simulink model "RoboBoat_SLAM_6_29"  (R2014a)
settings: Solver=FixedStepDiscrete  StartTime=0.0  StopTime=inf  FixedStep=.1  RelTol=1e-3
undefined symbols (not defined in the file): Com1, Com2, Com3, Com4, DiscIntNeverNeededParam, standard
libraries: xpcseriallib x29, visiontextngfix x25, simulink x21, slrtlib x7, speedgoatlib_IO102 x5, speedgoatlib x1
(part 4 of 6)

== system RoboBoat_SLAM_6_29/Main FSM/Obstacle Navigation1/GPS: Center/Approach ==
  Sensors : Inport
  RGB image : Inport  Port=2
  Enable : EnablePort
  Annotate Task : visiontextngfix/Insert Text  inputType=Obsolete  theText='GPS - Center: Approach - Distance: %f'  getTextLocFrom=Specify via dialog  textLoc=[10 70]  getTextColorFrom=Specify via dialog  textColor=[255 0 0]  getTextIntensityFrom=Specify via dialog  textIntensity=0  getTextOpacityFrom=Specify via dialog  textOpacity=1.0  dummyVar2=0  dummyVar3=0  dummyVar4=0  imagePorts=One multidimensional signal  isInputTransposed=off  fontFace=LucidaSansRegular  dummyVar1=0  blockFontSize=12  antiAliased=on
  Annotate Task2 : visiontextngfix/Insert Text  inputType=Obsolete  theText='Obst Nav Start'  getTextLocFrom=Specify via dialog  textLoc=[1 1]  getTextColorFrom=Specify via dialog  textColor=[0 0 0]  getTextIntensityFrom=Specify via dialog  textIntensity=0  getTextOpacityFrom=Specify via dialog  textOpacity=1.0  dummyVar2=0  dummyVar3=0  dummyVar4=0  imagePorts=One multidimensional signal  isInputTransposed=off  fontFace=LucidaSansRegular  dummyVar1=0  blockFontSize=12  antiAliased=on
  Bus Selector : BusSelector  OutputSignals=Serial In.GPS.latitude,Serial In.GPS.longitude
  Compare To Constant : simulink/Logic and Bit Operations/Compare To Constant  relop=<=  const=5  OutDataTypeStr=boolean
  Data Store Read : DataStoreRead  DataStoreName=obstNavStartGPS  SampleTime=0.1
  Data Type Conversion : DataTypeConversion  OutDataTypeStr=double
  Desired Heading and Distance : MATLAB Function  TreatAsAtomicUnit=on
  MATLAB Function : MATLAB Function  Commented=on  TreatAsAtomicUnit=on
  Output Heirarchy : Subsystem
  "Scope " : slrtlib/Displays and Logging/Scope   Commented=on  scopeno=1  scopetype=File  autostart=on  viewmode=Graphical redraw  formatstr='%15.6f'  grid=on  ylimits=[0,0]  nosamples=1200  noprepostsamples=0  interleave=1  triggermode=FreeRun  triggersignal=1  trigsignalfromport=off  triggerlevel=1  triggerslope=Either  triggerscope=1  triggersample=0  filename=ApprLog.dat  mode=Lazy  writesize=512  autorestart=off  dynamicfilemode=off  maxwritefilesize=512*1024^2
  Outputs : Outport
  wires:
  Sensors/1 -> Output Heirarchy/4(Sensors), Bus Selector/1  "Sensors"
  Data Store Read/1 -> Desired Heading and Distance/1(DesiredGPS)
  Bus Selector/1 -> Desired Heading and Distance/2(GPSLat)  "<latitude>"
  Bus Selector/2 -> Desired Heading and Distance/3(GPSLong)  "<longitude>"
  Desired Heading and Distance/2(DesiredHeading) -> Output Heirarchy/2(Desired Heading)
  Annotate Task/1 -> Output Heirarchy/3(Annotated Image)
  RGB image/1 -> Annotate Task2/1
  Output Heirarchy/1(Outputs) -> Outputs/1
  Annotate Task2/1 -> Annotate Task/1
  MATLAB Function/1(out) -> "Scope "/1
  Desired Heading and Distance/1(Distance) -> Compare To Constant/1, Annotate Task/2
  Data Type Conversion/1 -> Output Heirarchy/1(Finished)  "Task Finished"
  Compare To Constant/1 -> Data Type Conversion/1

== system RoboBoat_SLAM_6_29/Main FSM/Obstacle Navigation1/GPS: Center/Orient ==
  Sensors : Inport
  RGB image : Inport  Port=2
  Enable : EnablePort
  Annotate Task : visiontextngfix/Insert Text  inputType=Obsolete  theText='GPS - Center: Orient %f'  getTextLocFrom=Specify via dialog  textLoc=[10 70]  getTextColorFrom=Specify via dialog  textColor=[255 0 0]  getTextIntensityFrom=Specify via dialog  textIntensity=0  getTextOpacityFrom=Specify via dialog  textOpacity=1.0  dummyVar2=0  dummyVar3=0  dummyVar4=0  imagePorts=One multidimensional signal  isInputTransposed=off  fontFace=LucidaSansRegular  dummyVar1=0  blockFontSize=12  antiAliased=on
  Annotate Task1 : visiontextngfix/Insert Text  inputType=Obsolete  theText='Current Heading %f'  getTextLocFrom=Specify via dialog  textLoc=[10 40]  getTextColorFrom=Specify via dialog  textColor=[255 0 0]  getTextIntensityFrom=Specify via dialog  textIntensity=0  getTextOpacityFrom=Specify via dialog  textOpacity=1.0  dummyVar2=0  dummyVar3=0  dummyVar4=0  imagePorts=One multidimensional signal  isInputTransposed=off  fontFace=LucidaSansRegular  dummyVar1=0  blockFontSize=12  antiAliased=on
  Annotate Task2 : visiontextngfix/Insert Text  inputType=Obsolete  theText='Obst Nav Start'  getTextLocFrom=Specify via dialog  textLoc=[1 1]  getTextColorFrom=Specify via dialog  textColor=[0 0 0]  getTextIntensityFrom=Specify via dialog  textIntensity=0  getTextOpacityFrom=Specify via dialog  textOpacity=1.0  dummyVar2=0  dummyVar3=0  dummyVar4=0  imagePorts=One multidimensional signal  isInputTransposed=off  fontFace=LucidaSansRegular  dummyVar1=0  blockFontSize=12  antiAliased=on
  Bus Selector : BusSelector  OutputSignals=Serial In.GPS.latitude,Serial In.GPS.longitude,Serial In.Compass.Heading
  Data Store Read : DataStoreRead  DataStoreName=obstNavStartGPS  SampleTime=0.1
  Desired Heading : MATLAB Function  TreatAsAtomicUnit=on
  Output Heirarchy1 : Subsystem
  Within Range : MATLAB Function  TreatAsAtomicUnit=on
  Outputs : Outport
  Finished : Outport  Port=2
  wires:
  Sensors/1 -> Output Heirarchy1/3(Sensors), Bus Selector/1  "Sensors"
  Data Store Read/1 -> Desired Heading/1(DesiredGPS)
  Bus Selector/1 -> Desired Heading/2(GPSLat)  "<latitude>"
  Bus Selector/2 -> Desired Heading/3(GPSLong)  "<longitude>"
  Desired Heading/1(DesiredHeading) -> Output Heirarchy1/2(Desired Heading), Annotate Task/2, Within Range/1(DesiredHeading)
  Bus Selector/3 -> Annotate Task1/2, Within Range/2(Compass)  "<Heading>"
  Within Range/1(Finished) -> Finished/1
  RGB image/1 -> Annotate Task2/1
  Output Heirarchy1/1(Outputs) -> Outputs/1
  Annotate Task/1 -> Annotate Task1/1
  Annotate Task1/1 -> Output Heirarchy1/1(Annotated Image)
  Annotate Task2/1 -> Annotate Task/1

== system RoboBoat_SLAM_6_29/Main FSM/Obstacle Navigation1/GPS: Center/Output Reassign ==
  Outputs in : Inport
  Bus Assignment : BusAssignment  AssignedSignals=Task Finished
  Bus Selector : BusSelector  OutputSignals=Task Finished
  Constant : Constant  Value=0
  Outputs : Outport
  Finished : Outport  Port=2
  wires:
  Outputs in/1 -> Bus Assignment/1, Bus Selector/1
  Bus Selector/1 -> Finished/1  "<Task Finished>"
  Bus Assignment/1 -> Outputs/1
  Constant/1 -> Bus Assignment/2

== system RoboBoat_SLAM_6_29/Main FSM/Obstacle Navigation1/Obstacle Navigation/Dodge ==
  Sensors : Inport
  RGB image : Inport  Port=2
  Enable : EnablePort  ShowOutputPort=on
  Bus Selector1 : BusSelector  OutputSignals=Serial In.Compass.Heading,Serial In.Buoy Info.Distance,Serial In.Buoy Info.Angle
  Constant : Constant  Value=0
  Constant1 : Constant  Value=2
  Data Store Write : DataStoreWrite  DataStoreName=dodgeStart
  Discrete-Time Integrator : DiscreteIntegrator  SampleTime=0.1  ICPrevOutput=DiscIntNeverNeededParam  ICPrevScaledInput=DiscIntNeverNeededParam
  Insert Text : visiontextngfix/Insert Text  inputType=Obsolete  theText='Dodge'  getTextLocFrom=Specify via dialog  textLoc=[1 1]  getTextColorFrom=Specify via dialog  textColor=[0 0 0]  getTextIntensityFrom=Specify via dialog  textIntensity=0  getTextOpacityFrom=Specify via dialog  textOpacity=1.0  dummyVar2=0  dummyVar3=0  dummyVar4=0  imagePorts=One multidimensional signal  isInputTransposed=off  fontFace=LucidaSansRegular  dummyVar1=0  blockFontSize=12  antiAliased=on
  Insert Text1 : visiontextngfix/Insert Text  inputType=Obsolete  theText='Obstacle Distance: %f'  getTextLocFrom=Specify via dialog  textLoc=[10 70]  getTextColorFrom=Specify via dialog  textColor=[255 0 0]  getTextIntensityFrom=Specify via dialog  textIntensity=0  getTextOpacityFrom=Specify via dialog  textOpacity=1.0  dummyVar2=0  dummyVar3=0  dummyVar4=0  imagePorts=One multidimensional signal  isInputTransposed=off  fontFace=LucidaSansRegular  dummyVar1=0  blockFontSize=12  antiAliased=on
  Nav Logic : MATLAB Function  TreatAsAtomicUnit=on
  Output Heirarchy : Subsystem
  Unit Delay1 : UnitDelay  InitialCondition=1  SampleTime=-1
  Outputs : Outport
  Dodge Incomplete : Outport  Port=2
  wires:
  RGB image/1 -> Insert Text/1
  Sensors/1 -> Output Heirarchy/2(Sensors), Bus Selector1/1
  Bus Selector1/1 -> Nav Logic/1(CurrentHeading)  "<Heading>"
  Enable/1 -> Discrete-Time Integrator/1
  Discrete-Time Integrator/1 -> Nav Logic/4(Timer)
  Constant1/1 -> Nav Logic/5(Timeout)
  Nav Logic/4(DodgeIncomplete) -> Dodge Incomplete/1
  Insert Text/1 -> Insert Text1/1
  Nav Logic/1(ObstDist) -> Insert Text1/2
  Nav Logic/2(RPM) -> Output Heirarchy/3(RPM)
  Nav Logic/3(DesiredHeading) -> Output Heirarchy/4(Desired Heading)
  Output Heirarchy/1(Outputs) -> Outputs/1
  Constant/1 -> Unit Delay1/1
  Unit Delay1/1 -> Data Store Write/1
  Insert Text1/1 -> Output Heirarchy/1(Annotated Image)
  Bus Selector1/2 -> Nav Logic/2(Dist)  "<Distance>"
  Bus Selector1/3 -> Nav Logic/3(Ang)  "<Angle>"

== system RoboBoat_SLAM_6_29/Main FSM/Obstacle Navigation1/Obstacle Navigation/GPS: Bee Line ==
  Sensors : Inport
  RGB image : Inport  Port=2
  Enable : EnablePort
  Approach : Subsystem  TreatAsAtomicUnit=on
  Data Store Write : DataStoreWrite  DataStoreName=dodgeStart
  GPS Enabler : MATLAB Function  TreatAsAtomicUnit=on
  GPS Selector : MultiPortSwitch  Inputs=2
  Orient : Subsystem  TreatAsAtomicUnit=on
  Unit Delay : UnitDelay  SampleTime=-1
  Unit Delay1 : UnitDelay  SampleTime=-1
  Outputs : Outport
  wires:
  Sensors/1 -> Orient/1(Sensors), Approach/1(Sensors)
  GPS Enabler/2(OrientEnable) -> Orient/Enable
  GPS Enabler/3(ApproachEnable) -> Approach/Enable
  Orient/2(Finished) -> Unit Delay/1
  Orient/1(Outputs) -> GPS Selector/2
  Approach/1(Outputs) -> GPS Selector/3
  GPS Enabler/1(GPSMode) -> GPS Selector/1
  Unit Delay/1 -> GPS Enabler/1(Finished)
  RGB image/1 -> Orient/2(RGB image), Approach/2(RGB image)
  Approach/2(Dodge Start) -> Unit Delay1/1
  Unit Delay1/1 -> Data Store Write/1
  GPS Selector/1 -> Outputs/1

== system RoboBoat_SLAM_6_29/Main FSM/Obstacle Navigation1/Obstacle Navigation/Output Reassign ==
  Outputs in : Inport
  Bus Assignment : BusAssignment  AssignedSignals=Task Finished
  Bus Selector : BusSelector  OutputSignals=Task Finished
  Constant : Constant  Value=0
  Outputs : Outport
  Finished : Outport  Port=2
  wires:
  Outputs in/1 -> Bus Assignment/1, Bus Selector/1
  Bus Selector/1 -> Finished/1  "<Task Finished>"
  Bus Assignment/1 -> Outputs/1
  Constant/1 -> Bus Assignment/2

== system RoboBoat_SLAM_6_29/Main FSM/SLAM/Models for prediction/Model1 ==
  X : Inport
  Y : Inport  Port=2
  Psi : Inport  Port=3
  Nav Messages : Inport  Port=4
  Bus Creator : BusCreator  Inputs=3
  Bus Selector : BusSelector  OutputSignals=IMU.Velocity.u,IMU.Velocity.v,IMU.Rate of Turn.GyrZ,Thrust.PortPow,Thrust.StbdPow
  Model : ModelReference  ModelNameDialog=SeaCat_Dynamic_Model.slx  SimulationMode=Normal  ModelReferenceVersion=1.2137  CopyOfModelName=SeaCat_Dynamic_Model.slx  DefaultDataLogging=on
  No Azimuth : Constant  Value=0
  NEyaw : Outport
  wires:
  Nav Messages/1 -> Bus Selector/1
  X/1 -> Model/1
  Y/1 -> Model/2
  Psi/1 -> Model/3
  Bus Selector/1 -> Model/4  "<u>"
  Bus Selector/2 -> Model/5  "<v>"
  Bus Selector/3 -> Model/6  "<GyrZ>"
  Bus Selector/4 -> Model/7  "<PortPow>"
  Bus Selector/5 -> Model/9  "<StbdPow>"
  No Azimuth/1 -> Model/8, Model/10
  Model/1 -> Bus Creator/1  "N"
  Model/3 -> Bus Creator/3  "yaw"
  Model/2 -> Bus Creator/2  "E"
  Bus Creator/1 -> NEyaw/1

== system RoboBoat_SLAM_6_29/Main FSM/SLAM/Models for prediction/Model10 ==
  X : Inport
  Y : Inport  Port=2
  Psi : Inport  Port=3
  Nav Messages : Inport  Port=4
  Bus Creator : BusCreator  Inputs=3
  Bus Selector : BusSelector  OutputSignals=IMU.Velocity.u,IMU.Velocity.v,IMU.Rate of Turn.GyrZ,Thrust.PortPow,Thrust.StbdPow
  Model : ModelReference  ModelNameDialog=SeaCat_Dynamic_Model.slx  SimulationMode=Normal  ModelReferenceVersion=1.2137  CopyOfModelName=SeaCat_Dynamic_Model.slx  DefaultDataLogging=on
  No Azimuth : Constant  Value=0
  NEyaw : Outport
  wires:
  Nav Messages/1 -> Bus Selector/1
  X/1 -> Model/1
  Y/1 -> Model/2
  Psi/1 -> Model/3
  Bus Selector/1 -> Model/4  "<u>"
  Bus Selector/2 -> Model/5  "<v>"
  Bus Selector/3 -> Model/6  "<GyrZ>"
  Bus Selector/4 -> Model/7  "<PortPow>"
  Bus Selector/5 -> Model/9  "<StbdPow>"
  No Azimuth/1 -> Model/8, Model/10
  Model/1 -> Bus Creator/1  "N"
  Model/3 -> Bus Creator/3  "yaw"
  Model/2 -> Bus Creator/2  "E"
  Bus Creator/1 -> NEyaw/1

== system RoboBoat_SLAM_6_29/Main FSM/SLAM/Models for prediction/Model11 ==
  X : Inport
  Y : Inport  Port=2
  Psi : Inport  Port=3
  Nav Messages : Inport  Port=4
  Bus Creator : BusCreator  Inputs=3
  Bus Selector : BusSelector  OutputSignals=IMU.Velocity.u,IMU.Velocity.v,IMU.Rate of Turn.GyrZ,Thrust.PortPow,Thrust.StbdPow
  Model : ModelReference  ModelNameDialog=SeaCat_Dynamic_Model.slx  SimulationMode=Normal  ModelReferenceVersion=1.2137  CopyOfModelName=SeaCat_Dynamic_Model.slx  DefaultDataLogging=on
  No Azimuth : Constant  Value=0
  NEyaw : Outport
  wires:
  Nav Messages/1 -> Bus Selector/1
  X/1 -> Model/1
  Y/1 -> Model/2
  Psi/1 -> Model/3
  Bus Selector/1 -> Model/4  "<u>"
  Bus Selector/2 -> Model/5  "<v>"
  Bus Selector/3 -> Model/6  "<GyrZ>"
  Bus Selector/4 -> Model/7  "<PortPow>"
  Bus Selector/5 -> Model/9  "<StbdPow>"
  No Azimuth/1 -> Model/8, Model/10
  Model/1 -> Bus Creator/1  "N"
  Model/3 -> Bus Creator/3  "yaw"
  Model/2 -> Bus Creator/2  "E"
  Bus Creator/1 -> NEyaw/1

== system RoboBoat_SLAM_6_29/Main FSM/SLAM/Models for prediction/Model12 ==
  X : Inport
  Y : Inport  Port=2
  Psi : Inport  Port=3
  Nav Messages : Inport  Port=4
  Bus Creator : BusCreator  Inputs=3
  Bus Selector : BusSelector  OutputSignals=IMU.Velocity.u,IMU.Velocity.v,IMU.Rate of Turn.GyrZ,Thrust.PortPow,Thrust.StbdPow
  Model : ModelReference  ModelNameDialog=SeaCat_Dynamic_Model.slx  SimulationMode=Normal  ModelReferenceVersion=1.2137  CopyOfModelName=SeaCat_Dynamic_Model.slx  DefaultDataLogging=on
  No Azimuth : Constant  Value=0
  NEyaw : Outport
  wires:
  Nav Messages/1 -> Bus Selector/1
  X/1 -> Model/1
  Y/1 -> Model/2
  Psi/1 -> Model/3
  Bus Selector/1 -> Model/4  "<u>"
  Bus Selector/2 -> Model/5  "<v>"
  Bus Selector/3 -> Model/6  "<GyrZ>"
  Bus Selector/4 -> Model/7  "<PortPow>"
  Bus Selector/5 -> Model/9  "<StbdPow>"
  No Azimuth/1 -> Model/8, Model/10
  Model/1 -> Bus Creator/1  "N"
  Model/3 -> Bus Creator/3  "yaw"
  Model/2 -> Bus Creator/2  "E"
  Bus Creator/1 -> NEyaw/1

== system RoboBoat_SLAM_6_29/Main FSM/SLAM/Models for prediction/Model13 ==
  X : Inport
  Y : Inport  Port=2
  Psi : Inport  Port=3
  Nav Messages : Inport  Port=4
  Bus Creator : BusCreator  Inputs=3
  Bus Selector : BusSelector  OutputSignals=IMU.Velocity.u,IMU.Velocity.v,IMU.Rate of Turn.GyrZ,Thrust.PortPow,Thrust.StbdPow
  Model : ModelReference  ModelNameDialog=SeaCat_Dynamic_Model.slx  SimulationMode=Normal  ModelReferenceVersion=1.2137  CopyOfModelName=SeaCat_Dynamic_Model.slx  DefaultDataLogging=on
  No Azimuth : Constant  Value=0
  NEyaw : Outport
  wires:
  Nav Messages/1 -> Bus Selector/1
  X/1 -> Model/1
  Y/1 -> Model/2
  Psi/1 -> Model/3
  Bus Selector/1 -> Model/4  "<u>"
  Bus Selector/2 -> Model/5  "<v>"
  Bus Selector/3 -> Model/6  "<GyrZ>"
  Bus Selector/4 -> Model/7  "<PortPow>"
  Bus Selector/5 -> Model/9  "<StbdPow>"
  No Azimuth/1 -> Model/8, Model/10
  Model/1 -> Bus Creator/1  "N"
  Model/3 -> Bus Creator/3  "yaw"
  Model/2 -> Bus Creator/2  "E"
  Bus Creator/1 -> NEyaw/1

== system RoboBoat_SLAM_6_29/Main FSM/SLAM/Models for prediction/Model14 ==
  X : Inport
  Y : Inport  Port=2
  Psi : Inport  Port=3
  Nav Messages : Inport  Port=4
  Bus Creator : BusCreator  Inputs=3
  Bus Selector : BusSelector  OutputSignals=IMU.Velocity.u,IMU.Velocity.v,IMU.Rate of Turn.GyrZ,Thrust.PortPow,Thrust.StbdPow
  Model : ModelReference  ModelNameDialog=SeaCat_Dynamic_Model.slx  SimulationMode=Normal  ModelReferenceVersion=1.2137  CopyOfModelName=SeaCat_Dynamic_Model.slx  DefaultDataLogging=on
  No Azimuth : Constant  Value=0
  NEyaw : Outport
  wires:
  Nav Messages/1 -> Bus Selector/1
  X/1 -> Model/1
  Y/1 -> Model/2
  Psi/1 -> Model/3
  Bus Selector/1 -> Model/4  "<u>"
  Bus Selector/2 -> Model/5  "<v>"
  Bus Selector/3 -> Model/6  "<GyrZ>"
  Bus Selector/4 -> Model/7  "<PortPow>"
  Bus Selector/5 -> Model/9  "<StbdPow>"
  No Azimuth/1 -> Model/8, Model/10
  Model/1 -> Bus Creator/1  "N"
  Model/3 -> Bus Creator/3  "yaw"
  Model/2 -> Bus Creator/2  "E"
  Bus Creator/1 -> NEyaw/1

== system RoboBoat_SLAM_6_29/Main FSM/SLAM/Models for prediction/Model15 ==
  X : Inport
  Y : Inport  Port=2
  Psi : Inport  Port=3
  Nav Messages : Inport  Port=4
  Bus Creator : BusCreator  Inputs=3
  Bus Selector : BusSelector  OutputSignals=IMU.Velocity.u,IMU.Velocity.v,IMU.Rate of Turn.GyrZ,Thrust.PortPow,Thrust.StbdPow
  Model : ModelReference  ModelNameDialog=SeaCat_Dynamic_Model.slx  SimulationMode=Normal  ModelReferenceVersion=1.2137  CopyOfModelName=SeaCat_Dynamic_Model.slx  DefaultDataLogging=on
  No Azimuth : Constant  Value=0
  NEyaw : Outport
  wires:
  Nav Messages/1 -> Bus Selector/1
  X/1 -> Model/1
  Y/1 -> Model/2
  Psi/1 -> Model/3
  Bus Selector/1 -> Model/4  "<u>"
  Bus Selector/2 -> Model/5  "<v>"
  Bus Selector/3 -> Model/6  "<GyrZ>"
  Bus Selector/4 -> Model/7  "<PortPow>"
  Bus Selector/5 -> Model/9  "<StbdPow>"
  No Azimuth/1 -> Model/8, Model/10
  Model/1 -> Bus Creator/1  "N"
  Model/3 -> Bus Creator/3  "yaw"
  Model/2 -> Bus Creator/2  "E"
  Bus Creator/1 -> NEyaw/1

== system RoboBoat_SLAM_6_29/Main FSM/SLAM/Models for prediction/Model16 ==
  X : Inport
  Y : Inport  Port=2
  Psi : Inport  Port=3
  Nav Messages : Inport  Port=4
  Bus Creator : BusCreator  Inputs=3
  Bus Selector : BusSelector  OutputSignals=IMU.Velocity.u,IMU.Velocity.v,IMU.Rate of Turn.GyrZ,Thrust.PortPow,Thrust.StbdPow
  Model : ModelReference  ModelNameDialog=SeaCat_Dynamic_Model.slx  SimulationMode=Normal  ModelReferenceVersion=1.2137  CopyOfModelName=SeaCat_Dynamic_Model.slx  DefaultDataLogging=on
  No Azimuth : Constant  Value=0
  NEyaw : Outport
  wires:
  Nav Messages/1 -> Bus Selector/1
  X/1 -> Model/1
  Y/1 -> Model/2
  Psi/1 -> Model/3
  Bus Selector/1 -> Model/4  "<u>"
  Bus Selector/2 -> Model/5  "<v>"
  Bus Selector/3 -> Model/6  "<GyrZ>"
  Bus Selector/4 -> Model/7  "<PortPow>"
  Bus Selector/5 -> Model/9  "<StbdPow>"
  No Azimuth/1 -> Model/8, Model/10
  Model/1 -> Bus Creator/1  "N"
  Model/3 -> Bus Creator/3  "yaw"
  Model/2 -> Bus Creator/2  "E"
  Bus Creator/1 -> NEyaw/1

== system RoboBoat_SLAM_6_29/Main FSM/SLAM/Models for prediction/Model17 ==
  X : Inport
  Y : Inport  Port=2
  Psi : Inport  Port=3
  Nav Messages : Inport  Port=4
  Bus Creator : BusCreator  Inputs=3
  Bus Selector : BusSelector  OutputSignals=IMU.Velocity.u,IMU.Velocity.v,IMU.Rate of Turn.GyrZ,Thrust.PortPow,Thrust.StbdPow
  Model : ModelReference  ModelNameDialog=SeaCat_Dynamic_Model.slx  SimulationMode=Normal  ModelReferenceVersion=1.2137  CopyOfModelName=SeaCat_Dynamic_Model.slx  DefaultDataLogging=on
  No Azimuth : Constant  Value=0
  NEyaw : Outport
  wires:
  Nav Messages/1 -> Bus Selector/1
  X/1 -> Model/1
  Y/1 -> Model/2
  Psi/1 -> Model/3
  Bus Selector/1 -> Model/4  "<u>"
  Bus Selector/2 -> Model/5  "<v>"
  Bus Selector/3 -> Model/6  "<GyrZ>"
  Bus Selector/4 -> Model/7  "<PortPow>"
  Bus Selector/5 -> Model/9  "<StbdPow>"
  No Azimuth/1 -> Model/8, Model/10
  Model/1 -> Bus Creator/1  "N"
  Model/3 -> Bus Creator/3  "yaw"
  Model/2 -> Bus Creator/2  "E"
  Bus Creator/1 -> NEyaw/1

== system RoboBoat_SLAM_6_29/Main FSM/SLAM/Models for prediction/Model18 ==
  X : Inport
  Y : Inport  Port=2
  Psi : Inport  Port=3
  Nav Messages : Inport  Port=4
  Bus Creator : BusCreator  Inputs=3
  Bus Selector : BusSelector  OutputSignals=IMU.Velocity.u,IMU.Velocity.v,IMU.Rate of Turn.GyrZ,Thrust.PortPow,Thrust.StbdPow
  Model : ModelReference  ModelNameDialog=SeaCat_Dynamic_Model.slx  SimulationMode=Normal  ModelReferenceVersion=1.2137  CopyOfModelName=SeaCat_Dynamic_Model.slx  DefaultDataLogging=on
  No Azimuth : Constant  Value=0
  NEyaw : Outport
  wires:
  Nav Messages/1 -> Bus Selector/1
  X/1 -> Model/1
  Y/1 -> Model/2
  Psi/1 -> Model/3
  Bus Selector/1 -> Model/4  "<u>"
  Bus Selector/2 -> Model/5  "<v>"
  Bus Selector/3 -> Model/6  "<GyrZ>"
  Bus Selector/4 -> Model/7  "<PortPow>"
  Bus Selector/5 -> Model/9  "<StbdPow>"
  No Azimuth/1 -> Model/8, Model/10
  Model/1 -> Bus Creator/1  "N"
  Model/3 -> Bus Creator/3  "yaw"
  Model/2 -> Bus Creator/2  "E"
  Bus Creator/1 -> NEyaw/1

== system RoboBoat_SLAM_6_29/Main FSM/SLAM/Models for prediction/Model19 ==
  X : Inport
  Y : Inport  Port=2
  Psi : Inport  Port=3
  Nav Messages : Inport  Port=4
  Bus Creator : BusCreator  Inputs=3
  Bus Selector : BusSelector  OutputSignals=IMU.Velocity.u,IMU.Velocity.v,IMU.Rate of Turn.GyrZ,Thrust.PortPow,Thrust.StbdPow
  Model : ModelReference  ModelNameDialog=SeaCat_Dynamic_Model.slx  SimulationMode=Normal  ModelReferenceVersion=1.2137  CopyOfModelName=SeaCat_Dynamic_Model.slx  DefaultDataLogging=on
  No Azimuth : Constant  Value=0
  NEyaw : Outport
  wires:
  Nav Messages/1 -> Bus Selector/1
  X/1 -> Model/1
  Y/1 -> Model/2
  Psi/1 -> Model/3
  Bus Selector/1 -> Model/4  "<u>"
  Bus Selector/2 -> Model/5  "<v>"
  Bus Selector/3 -> Model/6  "<GyrZ>"
  Bus Selector/4 -> Model/7  "<PortPow>"
  Bus Selector/5 -> Model/9  "<StbdPow>"
  No Azimuth/1 -> Model/8, Model/10
  Model/1 -> Bus Creator/1  "N"
  Model/3 -> Bus Creator/3  "yaw"
  Model/2 -> Bus Creator/2  "E"
  Bus Creator/1 -> NEyaw/1

== system RoboBoat_SLAM_6_29/Main FSM/SLAM/Models for prediction/Model2 ==
  X : Inport
  Y : Inport  Port=2
  Psi : Inport  Port=3
  Nav Messages : Inport  Port=4
  Bus Creator : BusCreator  Inputs=3
  Bus Selector : BusSelector  OutputSignals=IMU.Velocity.u,IMU.Velocity.v,IMU.Rate of Turn.GyrZ,Thrust.PortPow,Thrust.StbdPow
  Model : ModelReference  ModelNameDialog=SeaCat_Dynamic_Model.slx  SimulationMode=Normal  ModelReferenceVersion=1.2137  CopyOfModelName=SeaCat_Dynamic_Model.slx  DefaultDataLogging=on
  No Azimuth : Constant  Value=0
  NEyaw : Outport
  wires:
  Nav Messages/1 -> Bus Selector/1
  X/1 -> Model/1
  Y/1 -> Model/2
  Psi/1 -> Model/3
  Bus Selector/1 -> Model/4  "<u>"
  Bus Selector/2 -> Model/5  "<v>"
  Bus Selector/3 -> Model/6  "<GyrZ>"
  Bus Selector/4 -> Model/7  "<PortPow>"
  Bus Selector/5 -> Model/9  "<StbdPow>"
  No Azimuth/1 -> Model/8, Model/10
  Model/1 -> Bus Creator/1  "N"
  Model/3 -> Bus Creator/3  "yaw"
  Model/2 -> Bus Creator/2  "E"
  Bus Creator/1 -> NEyaw/1

== system RoboBoat_SLAM_6_29/Main FSM/SLAM/Models for prediction/Model20 ==
  X : Inport
  Y : Inport  Port=2
  Psi : Inport  Port=3
  Nav Messages : Inport  Port=4
  Bus Creator : BusCreator  Inputs=3
  Bus Selector : BusSelector  OutputSignals=IMU.Velocity.u,IMU.Velocity.v,IMU.Rate of Turn.GyrZ,Thrust.PortPow,Thrust.StbdPow
  Model : ModelReference  ModelNameDialog=SeaCat_Dynamic_Model.slx  SimulationMode=Normal  ModelReferenceVersion=1.2137  CopyOfModelName=SeaCat_Dynamic_Model.slx  DefaultDataLogging=on
  No Azimuth : Constant  Value=0
  NEyaw : Outport
  wires:
  Nav Messages/1 -> Bus Selector/1
  X/1 -> Model/1
  Y/1 -> Model/2
  Psi/1 -> Model/3
  Bus Selector/1 -> Model/4  "<u>"
  Bus Selector/2 -> Model/5  "<v>"
  Bus Selector/3 -> Model/6  "<GyrZ>"
  Bus Selector/4 -> Model/7  "<PortPow>"
  Bus Selector/5 -> Model/9  "<StbdPow>"
  No Azimuth/1 -> Model/8, Model/10
  Model/1 -> Bus Creator/1  "N"
  Model/3 -> Bus Creator/3  "yaw"
  Model/2 -> Bus Creator/2  "E"
  Bus Creator/1 -> NEyaw/1

== system RoboBoat_SLAM_6_29/Main FSM/SLAM/Models for prediction/Model21 ==
  X : Inport
  Y : Inport  Port=2
  Psi : Inport  Port=3
  Nav Messages : Inport  Port=4
  Bus Creator : BusCreator  Inputs=3
  Bus Selector : BusSelector  OutputSignals=IMU.Velocity.u,IMU.Velocity.v,IMU.Rate of Turn.GyrZ,Thrust.PortPow,Thrust.StbdPow
  Model : ModelReference  ModelNameDialog=SeaCat_Dynamic_Model.slx  SimulationMode=Normal  ModelReferenceVersion=1.2137  CopyOfModelName=SeaCat_Dynamic_Model.slx  DefaultDataLogging=on
  No Azimuth : Constant  Value=0
  NEyaw : Outport
  wires:
  Nav Messages/1 -> Bus Selector/1
  X/1 -> Model/1
  Y/1 -> Model/2
  Psi/1 -> Model/3
  Bus Selector/1 -> Model/4  "<u>"
  Bus Selector/2 -> Model/5  "<v>"
  Bus Selector/3 -> Model/6  "<GyrZ>"
  Bus Selector/4 -> Model/7  "<PortPow>"
  Bus Selector/5 -> Model/9  "<StbdPow>"
  No Azimuth/1 -> Model/8, Model/10
  Model/1 -> Bus Creator/1  "N"
  Model/3 -> Bus Creator/3  "yaw"
  Model/2 -> Bus Creator/2  "E"
  Bus Creator/1 -> NEyaw/1

== system RoboBoat_SLAM_6_29/Main FSM/SLAM/Models for prediction/Model22 ==
  X : Inport
  Y : Inport  Port=2
  Psi : Inport  Port=3
  Nav Messages : Inport  Port=4
  Bus Creator : BusCreator  Inputs=3
  Bus Selector : BusSelector  OutputSignals=IMU.Velocity.u,IMU.Velocity.v,IMU.Rate of Turn.GyrZ,Thrust.PortPow,Thrust.StbdPow
  Model : ModelReference  ModelNameDialog=SeaCat_Dynamic_Model.slx  SimulationMode=Normal  ModelReferenceVersion=1.2137  CopyOfModelName=SeaCat_Dynamic_Model.slx  DefaultDataLogging=on
  No Azimuth : Constant  Value=0
  NEyaw : Outport
  wires:
  Nav Messages/1 -> Bus Selector/1
  X/1 -> Model/1
  Y/1 -> Model/2
  Psi/1 -> Model/3
  Bus Selector/1 -> Model/4  "<u>"
  Bus Selector/2 -> Model/5  "<v>"
  Bus Selector/3 -> Model/6  "<GyrZ>"
  Bus Selector/4 -> Model/7  "<PortPow>"
  Bus Selector/5 -> Model/9  "<StbdPow>"
  No Azimuth/1 -> Model/8, Model/10
  Model/1 -> Bus Creator/1  "N"
  Model/3 -> Bus Creator/3  "yaw"
  Model/2 -> Bus Creator/2  "E"
  Bus Creator/1 -> NEyaw/1

== system RoboBoat_SLAM_6_29/Main FSM/SLAM/Models for prediction/Model23 ==
  X : Inport
  Y : Inport  Port=2
  Psi : Inport  Port=3
  Nav Messages : Inport  Port=4
  Bus Creator : BusCreator  Inputs=3
  Bus Selector : BusSelector  OutputSignals=IMU.Velocity.u,IMU.Velocity.v,IMU.Rate of Turn.GyrZ,Thrust.PortPow,Thrust.StbdPow
  Model : ModelReference  ModelNameDialog=SeaCat_Dynamic_Model.slx  SimulationMode=Normal  ModelReferenceVersion=1.2137  CopyOfModelName=SeaCat_Dynamic_Model.slx  DefaultDataLogging=on
  No Azimuth : Constant  Value=0
  NEyaw : Outport
  wires:
  Nav Messages/1 -> Bus Selector/1
  X/1 -> Model/1
  Y/1 -> Model/2
  Psi/1 -> Model/3
  Bus Selector/1 -> Model/4  "<u>"
  Bus Selector/2 -> Model/5  "<v>"
  Bus Selector/3 -> Model/6  "<GyrZ>"
  Bus Selector/4 -> Model/7  "<PortPow>"
  Bus Selector/5 -> Model/9  "<StbdPow>"
  No Azimuth/1 -> Model/8, Model/10
  Model/1 -> Bus Creator/1  "N"
  Model/3 -> Bus Creator/3  "yaw"
  Model/2 -> Bus Creator/2  "E"
  Bus Creator/1 -> NEyaw/1

== system RoboBoat_SLAM_6_29/Main FSM/SLAM/Models for prediction/Model24 ==
  X : Inport
  Y : Inport  Port=2
  Psi : Inport  Port=3
  Nav Messages : Inport  Port=4
  Bus Creator : BusCreator  Inputs=3
  Bus Selector : BusSelector  OutputSignals=IMU.Velocity.u,IMU.Velocity.v,IMU.Rate of Turn.GyrZ,Thrust.PortPow,Thrust.StbdPow
  Model : ModelReference  ModelNameDialog=SeaCat_Dynamic_Model.slx  SimulationMode=Normal  ModelReferenceVersion=1.2137  CopyOfModelName=SeaCat_Dynamic_Model.slx  DefaultDataLogging=on
  No Azimuth : Constant  Value=0
  NEyaw : Outport
  wires:
  Nav Messages/1 -> Bus Selector/1
  X/1 -> Model/1
  Y/1 -> Model/2
  Psi/1 -> Model/3
  Bus Selector/1 -> Model/4  "<u>"
  Bus Selector/2 -> Model/5  "<v>"
  Bus Selector/3 -> Model/6  "<GyrZ>"
  Bus Selector/4 -> Model/7  "<PortPow>"
  Bus Selector/5 -> Model/9  "<StbdPow>"
  No Azimuth/1 -> Model/8, Model/10
  Model/1 -> Bus Creator/1  "N"
  Model/3 -> Bus Creator/3  "yaw"
  Model/2 -> Bus Creator/2  "E"
  Bus Creator/1 -> NEyaw/1

== system RoboBoat_SLAM_6_29/Main FSM/SLAM/Models for prediction/Model25 ==
  X : Inport
  Y : Inport  Port=2
  Psi : Inport  Port=3
  Nav Messages : Inport  Port=4
  Bus Creator : BusCreator  Inputs=3
  Bus Selector : BusSelector  OutputSignals=IMU.Velocity.u,IMU.Velocity.v,IMU.Rate of Turn.GyrZ,Thrust.PortPow,Thrust.StbdPow
  Model : ModelReference  ModelNameDialog=SeaCat_Dynamic_Model.slx  SimulationMode=Normal  ModelReferenceVersion=1.2137  CopyOfModelName=SeaCat_Dynamic_Model.slx  DefaultDataLogging=on
  No Azimuth : Constant  Value=0
  NEyaw : Outport
  wires:
  Nav Messages/1 -> Bus Selector/1
  X/1 -> Model/1
  Y/1 -> Model/2
  Psi/1 -> Model/3
  Bus Selector/1 -> Model/4  "<u>"
  Bus Selector/2 -> Model/5  "<v>"
  Bus Selector/3 -> Model/6  "<GyrZ>"
  Bus Selector/4 -> Model/7  "<PortPow>"
  Bus Selector/5 -> Model/9  "<StbdPow>"
  No Azimuth/1 -> Model/8, Model/10
  Model/1 -> Bus Creator/1  "N"
  Model/3 -> Bus Creator/3  "yaw"
  Model/2 -> Bus Creator/2  "E"
  Bus Creator/1 -> NEyaw/1

== system RoboBoat_SLAM_6_29/Main FSM/SLAM/Models for prediction/Model26 ==
  X : Inport
  Y : Inport  Port=2
  Psi : Inport  Port=3
  Nav Messages : Inport  Port=4
  Bus Creator : BusCreator  Inputs=3
  Bus Selector : BusSelector  OutputSignals=IMU.Velocity.u,IMU.Velocity.v,IMU.Rate of Turn.GyrZ,Thrust.PortPow,Thrust.StbdPow
  Model : ModelReference  ModelNameDialog=SeaCat_Dynamic_Model.slx  SimulationMode=Normal  ModelReferenceVersion=1.2137  CopyOfModelName=SeaCat_Dynamic_Model.slx  DefaultDataLogging=on
  No Azimuth : Constant  Value=0
  NEyaw : Outport
  wires:
  Nav Messages/1 -> Bus Selector/1
  X/1 -> Model/1
  Y/1 -> Model/2
  Psi/1 -> Model/3
  Bus Selector/1 -> Model/4  "<u>"
  Bus Selector/2 -> Model/5  "<v>"
  Bus Selector/3 -> Model/6  "<GyrZ>"
  Bus Selector/4 -> Model/7  "<PortPow>"
  Bus Selector/5 -> Model/9  "<StbdPow>"
  No Azimuth/1 -> Model/8, Model/10
  Model/1 -> Bus Creator/1  "N"
  Model/3 -> Bus Creator/3  "yaw"
  Model/2 -> Bus Creator/2  "E"
  Bus Creator/1 -> NEyaw/1

== system RoboBoat_SLAM_6_29/Main FSM/SLAM/Models for prediction/Model27 ==
  X : Inport
  Y : Inport  Port=2
  Psi : Inport  Port=3
  Nav Messages : Inport  Port=4
  Bus Creator : BusCreator  Inputs=3
  Bus Selector : BusSelector  OutputSignals=IMU.Velocity.u,IMU.Velocity.v,IMU.Rate of Turn.GyrZ,Thrust.PortPow,Thrust.StbdPow
  Model : ModelReference  ModelNameDialog=SeaCat_Dynamic_Model.slx  SimulationMode=Normal  ModelReferenceVersion=1.2137  CopyOfModelName=SeaCat_Dynamic_Model.slx  DefaultDataLogging=on
  No Azimuth : Constant  Value=0
  NEyaw : Outport
  wires:
  Nav Messages/1 -> Bus Selector/1
  X/1 -> Model/1
  Y/1 -> Model/2
  Psi/1 -> Model/3
  Bus Selector/1 -> Model/4  "<u>"
  Bus Selector/2 -> Model/5  "<v>"
  Bus Selector/3 -> Model/6  "<GyrZ>"
  Bus Selector/4 -> Model/7  "<PortPow>"
  Bus Selector/5 -> Model/9  "<StbdPow>"
  No Azimuth/1 -> Model/8, Model/10
  Model/1 -> Bus Creator/1  "N"
  Model/3 -> Bus Creator/3  "yaw"
  Model/2 -> Bus Creator/2  "E"
  Bus Creator/1 -> NEyaw/1

== system RoboBoat_SLAM_6_29/Main FSM/SLAM/Models for prediction/Model28 ==
  X : Inport
  Y : Inport  Port=2
  Psi : Inport  Port=3
  Nav Messages : Inport  Port=4
  Bus Creator : BusCreator  Inputs=3
  Bus Selector : BusSelector  OutputSignals=IMU.Velocity.u,IMU.Velocity.v,IMU.Rate of Turn.GyrZ,Thrust.PortPow,Thrust.StbdPow
  Model : ModelReference  ModelNameDialog=SeaCat_Dynamic_Model.slx  SimulationMode=Normal  ModelReferenceVersion=1.2137  CopyOfModelName=SeaCat_Dynamic_Model.slx  DefaultDataLogging=on
  No Azimuth : Constant  Value=0
  NEyaw : Outport
  wires:
  Nav Messages/1 -> Bus Selector/1
  X/1 -> Model/1
  Y/1 -> Model/2
  Psi/1 -> Model/3
  Bus Selector/1 -> Model/4  "<u>"
  Bus Selector/2 -> Model/5  "<v>"
  Bus Selector/3 -> Model/6  "<GyrZ>"
  Bus Selector/4 -> Model/7  "<PortPow>"
  Bus Selector/5 -> Model/9  "<StbdPow>"
  No Azimuth/1 -> Model/8, Model/10
  Model/1 -> Bus Creator/1  "N"
  Model/3 -> Bus Creator/3  "yaw"
  Model/2 -> Bus Creator/2  "E"
  Bus Creator/1 -> NEyaw/1

== system RoboBoat_SLAM_6_29/Main FSM/SLAM/Models for prediction/Model29 ==
  X : Inport
  Y : Inport  Port=2
  Psi : Inport  Port=3
  Nav Messages : Inport  Port=4
  Bus Creator : BusCreator  Inputs=3
  Bus Selector : BusSelector  OutputSignals=IMU.Velocity.u,IMU.Velocity.v,IMU.Rate of Turn.GyrZ,Thrust.PortPow,Thrust.StbdPow
  Model : ModelReference  ModelNameDialog=SeaCat_Dynamic_Model.slx  SimulationMode=Normal  ModelReferenceVersion=1.2137  CopyOfModelName=SeaCat_Dynamic_Model.slx  DefaultDataLogging=on
  No Azimuth : Constant  Value=0
  NEyaw : Outport
  wires:
  Nav Messages/1 -> Bus Selector/1
  X/1 -> Model/1
  Y/1 -> Model/2
  Psi/1 -> Model/3
  Bus Selector/1 -> Model/4  "<u>"
  Bus Selector/2 -> Model/5  "<v>"
  Bus Selector/3 -> Model/6  "<GyrZ>"
  Bus Selector/4 -> Model/7  "<PortPow>"
  Bus Selector/5 -> Model/9  "<StbdPow>"
  No Azimuth/1 -> Model/8, Model/10
  Model/1 -> Bus Creator/1  "N"
  Model/3 -> Bus Creator/3  "yaw"
  Model/2 -> Bus Creator/2  "E"
  Bus Creator/1 -> NEyaw/1

== system RoboBoat_SLAM_6_29/Main FSM/SLAM/Models for prediction/Model3 ==
  X : Inport
  Y : Inport  Port=2
  Psi : Inport  Port=3
  Nav Messages : Inport  Port=4
  Bus Creator : BusCreator  Inputs=3
  Bus Selector : BusSelector  OutputSignals=IMU.Velocity.u,IMU.Velocity.v,IMU.Rate of Turn.GyrZ,Thrust.PortPow,Thrust.StbdPow
  Model : ModelReference  ModelNameDialog=SeaCat_Dynamic_Model.slx  SimulationMode=Normal  ModelReferenceVersion=1.2137  CopyOfModelName=SeaCat_Dynamic_Model.slx  DefaultDataLogging=on
  No Azimuth : Constant  Value=0
  NEyaw : Outport
  wires:
  Nav Messages/1 -> Bus Selector/1
  X/1 -> Model/1
  Y/1 -> Model/2
  Psi/1 -> Model/3
  Bus Selector/1 -> Model/4  "<u>"
  Bus Selector/2 -> Model/5  "<v>"
  Bus Selector/3 -> Model/6  "<GyrZ>"
  Bus Selector/4 -> Model/7  "<PortPow>"
  Bus Selector/5 -> Model/9  "<StbdPow>"
  No Azimuth/1 -> Model/8, Model/10
  Model/1 -> Bus Creator/1  "N"
  Model/3 -> Bus Creator/3  "yaw"
  Model/2 -> Bus Creator/2  "E"
  Bus Creator/1 -> NEyaw/1

== system RoboBoat_SLAM_6_29/Main FSM/SLAM/Models for prediction/Model30 ==
  X : Inport
  Y : Inport  Port=2
  Psi : Inport  Port=3
  Nav Messages : Inport  Port=4
  Bus Creator : BusCreator  Inputs=3
  Bus Selector : BusSelector  OutputSignals=IMU.Velocity.u,IMU.Velocity.v,IMU.Rate of Turn.GyrZ,Thrust.PortPow,Thrust.StbdPow
  Model : ModelReference  ModelNameDialog=SeaCat_Dynamic_Model.slx  SimulationMode=Normal  ModelReferenceVersion=1.2137  CopyOfModelName=SeaCat_Dynamic_Model.slx  DefaultDataLogging=on
  No Azimuth : Constant  Value=0
  NEyaw : Outport
  wires:
  Nav Messages/1 -> Bus Selector/1
  X/1 -> Model/1
  Y/1 -> Model/2
  Psi/1 -> Model/3
  Bus Selector/1 -> Model/4  "<u>"
  Bus Selector/2 -> Model/5  "<v>"
  Bus Selector/3 -> Model/6  "<GyrZ>"
  Bus Selector/4 -> Model/7  "<PortPow>"
  Bus Selector/5 -> Model/9  "<StbdPow>"
  No Azimuth/1 -> Model/8, Model/10
  Model/1 -> Bus Creator/1  "N"
  Model/3 -> Bus Creator/3  "yaw"
  Model/2 -> Bus Creator/2  "E"
  Bus Creator/1 -> NEyaw/1

== system RoboBoat_SLAM_6_29/Main FSM/SLAM/Models for prediction/Model31 ==
  X : Inport
  Y : Inport  Port=2
  Psi : Inport  Port=3
  Nav Messages : Inport  Port=4
  Bus Creator : BusCreator  Inputs=3
  Bus Selector : BusSelector  OutputSignals=IMU.Velocity.u,IMU.Velocity.v,IMU.Rate of Turn.GyrZ,Thrust.PortPow,Thrust.StbdPow
  Model : ModelReference  ModelNameDialog=SeaCat_Dynamic_Model.slx  SimulationMode=Normal  ModelReferenceVersion=1.2137  CopyOfModelName=SeaCat_Dynamic_Model.slx  DefaultDataLogging=on
  No Azimuth : Constant  Value=0
  NEyaw : Outport
  wires:
  Nav Messages/1 -> Bus Selector/1
  X/1 -> Model/1
  Y/1 -> Model/2
  Psi/1 -> Model/3
  Bus Selector/1 -> Model/4  "<u>"
  Bus Selector/2 -> Model/5  "<v>"
  Bus Selector/3 -> Model/6  "<GyrZ>"
  Bus Selector/4 -> Model/7  "<PortPow>"
  Bus Selector/5 -> Model/9  "<StbdPow>"
  No Azimuth/1 -> Model/8, Model/10
  Model/1 -> Bus Creator/1  "N"
  Model/3 -> Bus Creator/3  "yaw"
  Model/2 -> Bus Creator/2  "E"
  Bus Creator/1 -> NEyaw/1

== system RoboBoat_SLAM_6_29/Main FSM/SLAM/Models for prediction/Model32 ==
  X : Inport
  Y : Inport  Port=2
  Psi : Inport  Port=3
  Nav Messages : Inport  Port=4
  Bus Creator : BusCreator  Inputs=3
  Bus Selector : BusSelector  OutputSignals=IMU.Velocity.u,IMU.Velocity.v,IMU.Rate of Turn.GyrZ,Thrust.PortPow,Thrust.StbdPow
  Model : ModelReference  ModelNameDialog=SeaCat_Dynamic_Model.slx  SimulationMode=Normal  ModelReferenceVersion=1.2137  CopyOfModelName=SeaCat_Dynamic_Model.slx  DefaultDataLogging=on
  No Azimuth : Constant  Value=0
  NEyaw : Outport
  wires:
  Nav Messages/1 -> Bus Selector/1
  X/1 -> Model/1
  Y/1 -> Model/2
  Psi/1 -> Model/3
  Bus Selector/1 -> Model/4  "<u>"
  Bus Selector/2 -> Model/5  "<v>"
  Bus Selector/3 -> Model/6  "<GyrZ>"
  Bus Selector/4 -> Model/7  "<PortPow>"
  Bus Selector/5 -> Model/9  "<StbdPow>"
  No Azimuth/1 -> Model/8, Model/10
  Model/1 -> Bus Creator/1  "N"
  Model/3 -> Bus Creator/3  "yaw"
  Model/2 -> Bus Creator/2  "E"
  Bus Creator/1 -> NEyaw/1

== system RoboBoat_SLAM_6_29/Main FSM/SLAM/Models for prediction/Model33 ==
  X : Inport
  Y : Inport  Port=2
  Psi : Inport  Port=3
  Nav Messages : Inport  Port=4
  Bus Creator : BusCreator  Inputs=3
  Bus Selector : BusSelector  OutputSignals=IMU.Velocity.u,IMU.Velocity.v,IMU.Rate of Turn.GyrZ,Thrust.PortPow,Thrust.StbdPow
  Model : ModelReference  ModelNameDialog=SeaCat_Dynamic_Model.slx  SimulationMode=Normal  ModelReferenceVersion=1.2137  CopyOfModelName=SeaCat_Dynamic_Model.slx  DefaultDataLogging=on
  No Azimuth : Constant  Value=0
  NEyaw : Outport
  wires:
  Nav Messages/1 -> Bus Selector/1
  X/1 -> Model/1
  Y/1 -> Model/2
  Psi/1 -> Model/3
  Bus Selector/1 -> Model/4  "<u>"
  Bus Selector/2 -> Model/5  "<v>"
  Bus Selector/3 -> Model/6  "<GyrZ>"
  Bus Selector/4 -> Model/7  "<PortPow>"
  Bus Selector/5 -> Model/9  "<StbdPow>"
  No Azimuth/1 -> Model/8, Model/10
  Model/1 -> Bus Creator/1  "N"
  Model/3 -> Bus Creator/3  "yaw"
  Model/2 -> Bus Creator/2  "E"
  Bus Creator/1 -> NEyaw/1

== system RoboBoat_SLAM_6_29/Main FSM/SLAM/Models for prediction/Model34 ==
  X : Inport
  Y : Inport  Port=2
  Psi : Inport  Port=3
  Nav Messages : Inport  Port=4
  Bus Creator : BusCreator  Inputs=3
  Bus Selector : BusSelector  OutputSignals=IMU.Velocity.u,IMU.Velocity.v,IMU.Rate of Turn.GyrZ,Thrust.PortPow,Thrust.StbdPow
  Model : ModelReference  ModelNameDialog=SeaCat_Dynamic_Model.slx  SimulationMode=Normal  ModelReferenceVersion=1.2137  CopyOfModelName=SeaCat_Dynamic_Model.slx  DefaultDataLogging=on
  No Azimuth : Constant  Value=0
  NEyaw : Outport
  wires:
  Nav Messages/1 -> Bus Selector/1
  X/1 -> Model/1
  Y/1 -> Model/2
  Psi/1 -> Model/3
  Bus Selector/1 -> Model/4  "<u>"
  Bus Selector/2 -> Model/5  "<v>"
  Bus Selector/3 -> Model/6  "<GyrZ>"
  Bus Selector/4 -> Model/7  "<PortPow>"
  Bus Selector/5 -> Model/9  "<StbdPow>"
  No Azimuth/1 -> Model/8, Model/10
  Model/1 -> Bus Creator/1  "N"
  Model/3 -> Bus Creator/3  "yaw"
  Model/2 -> Bus Creator/2  "E"
  Bus Creator/1 -> NEyaw/1

== system RoboBoat_SLAM_6_29/Main FSM/SLAM/Models for prediction/Model35 ==
  X : Inport
  Y : Inport  Port=2
  Psi : Inport  Port=3
  Nav Messages : Inport  Port=4
  Bus Creator : BusCreator  Inputs=3
  Bus Selector : BusSelector  OutputSignals=IMU.Velocity.u,IMU.Velocity.v,IMU.Rate of Turn.GyrZ,Thrust.PortPow,Thrust.StbdPow
  Model : ModelReference  ModelNameDialog=SeaCat_Dynamic_Model.slx  SimulationMode=Normal  ModelReferenceVersion=1.2137  CopyOfModelName=SeaCat_Dynamic_Model.slx  DefaultDataLogging=on
  No Azimuth : Constant  Value=0
  NEyaw : Outport
  wires:
  Nav Messages/1 -> Bus Selector/1
  X/1 -> Model/1
  Y/1 -> Model/2
  Psi/1 -> Model/3
  Bus Selector/1 -> Model/4  "<u>"
  Bus Selector/2 -> Model/5  "<v>"
  Bus Selector/3 -> Model/6  "<GyrZ>"
  Bus Selector/4 -> Model/7  "<PortPow>"
  Bus Selector/5 -> Model/9  "<StbdPow>"
  No Azimuth/1 -> Model/8, Model/10
  Model/1 -> Bus Creator/1  "N"
  Model/3 -> Bus Creator/3  "yaw"
  Model/2 -> Bus Creator/2  "E"
  Bus Creator/1 -> NEyaw/1

== system RoboBoat_SLAM_6_29/Main FSM/SLAM/Models for prediction/Model36 ==
  X : Inport
  Y : Inport  Port=2
  Psi : Inport  Port=3
  Nav Messages : Inport  Port=4
  Bus Creator : BusCreator  Inputs=3
  Bus Selector : BusSelector  OutputSignals=IMU.Velocity.u,IMU.Velocity.v,IMU.Rate of Turn.GyrZ,Thrust.PortPow,Thrust.StbdPow
  Model : ModelReference  ModelNameDialog=SeaCat_Dynamic_Model.slx  SimulationMode=Normal  ModelReferenceVersion=1.2137  CopyOfModelName=SeaCat_Dynamic_Model.slx  DefaultDataLogging=on
  No Azimuth : Constant  Value=0
  NEyaw : Outport
  wires:
  Nav Messages/1 -> Bus Selector/1
  X/1 -> Model/1
  Y/1 -> Model/2
  Psi/1 -> Model/3
  Bus Selector/1 -> Model/4  "<u>"
  Bus Selector/2 -> Model/5  "<v>"
  Bus Selector/3 -> Model/6  "<GyrZ>"
  Bus Selector/4 -> Model/7  "<PortPow>"
  Bus Selector/5 -> Model/9  "<StbdPow>"
  No Azimuth/1 -> Model/8, Model/10
  Model/1 -> Bus Creator/1  "N"
  Model/3 -> Bus Creator/3  "yaw"
  Model/2 -> Bus Creator/2  "E"
  Bus Creator/1 -> NEyaw/1

== matlab function RoboBoat_SLAM_6_29/Main FSM/Obstacle Navigation1/Exit Gate/Gate 1 (Red & White)/Distance ==
  data: Distance output; DesiredGPS input; GPSLat input; GPSLong input
function Distance  = DistCalc(DesiredGPS, GPSLat, GPSLong)

%Written by Anderson Lebbad on July 22, 2013
%Last Edited:

%Orients the boat towards a target GPS point before approaching it.
%This is done to keep the approach angle minimal, so the approach
%algorithm does not circle the target and never reach it.

%Parse input GPS and convert angles to radians
CurLat = (floor(GPSLat/100)+mod(GPSLat,100)/60)*pi/180;
CurLong = (floor(GPSLong/100)+mod(GPSLong,100)/60)*pi/180;
DesLat = (floor(DesiredGPS(1)/100)+mod(DesiredGPS(1),100)/60)*pi/180;
DesLong = (floor(DesiredGPS(2)/100)+mod(DesiredGPS(2),100)/60)*pi/180;
%Difference between lats and longs
DiffLat = DesLat - CurLat;
MidLat = cos((CurLat + DesLat)/2);
DiffLong = DesLong - CurLong;
%Radius of the earth in meters
R = 6378137;

%Calculate distance using the great-circle distance formula
%Formula documented here:
%   http://www.movable-type.co.uk/scripts/latlong.html
% a = sin(DiffLat/2)^2+sin(DiffLong/2)^2*cos(CurLat)*cos(DesLat);
% c = 2*atan2(sqrt(a), sqrt(1-a));
% Distance = R*c;

%Calculating distance using Pythagora's
a = DiffLong*MidLat;
b = DiffLat;
Distance = R*sqrt(a^2+b^2);

== matlab function RoboBoat_SLAM_6_29/Main FSM/Obstacle Navigation1/Exit Gate/Gate 2 (White & White)/MATLAB Function ==
  data: Prob input; RPM output; ColorID input; Dist input; Ang input; CurrentHeading input; GPSLat input; GPSLong input; Timer input; DesiredHeading output; gateGPS output
function [RPM,DesiredHeading,gateGPS] = navigation(Prob,ColorID,Dist,Ang,CurrentHeading,GPSLat,GPSLong,Timer)

% Function performs one buoy navigation through the start speed gates. If
% no buoys are found by the LIDAR/Vision assembly then an incremented
% turning algorithm is executed to turn by 10 degrees per increment up to 
% 90 degrees either way of the inital heading

% Written by Edward Zhu


persistent LockHeading TimeLastFound Counter Turn TurnInc gateLat gateLong

if isempty(LockHeading) && isempty(TimeLastFound) && isempty(Counter) && isempty(Turn) && isempty(TurnInc)
    LockHeading = CurrentHeading;
    TimeLastFound = 0;
    Counter = 0;
    TurnInc = 30;
    Turn = TurnInc;
    gateLat = 0;
    gateLong = 0;
end
Distance = Dist/100;
BoatWidth = 0.75;
Buffer = atan(2*BoatWidth/Distance);

RedOffset = Ang + Buffer;
WhiteOffset = Ang - Buffer;

R = 6378137;

CurLat = (floor(GPSLat/100)+mod(GPSLat,100)/60)*pi/180;
CurLong = (ceil(GPSLong/100)-mod(-GPSLong,100)/60)*pi/180;

gateHeading = (mod(CurrentHeading - Ang, 360))*pi/180;

if ColorID == 1 && Prob > 0.9
    DesiredHeading = mod(CurrentHeading - RedOffset, 360);
    RPM = 2000;
    GateFound = 1;
    TimeLastFound = Timer;
    gateLat =  asin(sin(CurLat)*cos(Distance/R) + cos(CurLat)*sin(Distance/R)*cos(gateHeading))*180/pi;
    gateLong = (CurLong + atan2(sin(gateHeading)*sin(Distance/R)*cos(CurLat),cos(Distance/R)-sin(CurLat)*sin(gateLat)))*180/pi;
elseif ColorID == 2 && Prob > 0.9
    DesiredHeading = mod(CurrentHeading - WhiteOffset, 360);
    RPM = 2000;
    GateFound = 1;
    TimeLastFound = Timer;
    gateLat =  asin(sin(CurLat)*cos(Distance/R) + cos(CurLat)*sin(Distance/R)*cos(gateHeading))*180/pi;
    gateLong = (CurLong + atan2(sin(gateHeading)*sin(Distance/R)*cos(CurLat),cos(Distance/R)-sin(CurLat)*sin(gateLat)))*180/pi;
else
    DesiredHeading = CurrentHeading;
    RPM = 0;
    GateFound = 0;
end

gateGPS = [gateLat gateLong];
TimeNoBuoys = Timer - TimeLastFound;

if GateFound == 0 && TimeNoBuoys > 15
    RPM = 0;
    DesiredHeading = mod(LockHeading - Turn, 360);
    HeadingDiff = DesiredHeading - CurrentHeading;
    gateGPS = [gateLat gateLong];
    
    if HeadingDiff > 180
        HeadingDiff = HeadingDiff - 360;
    elseif HeadingDiff < -180
        HeadingDiff = HeadingDiff + 360;
    end
    
    if HeadingDiff < 3
        Counter = Counter + 1;
    else
        Counter = 0;
    end
    
    if Counter >= 15
        Turn = Turn + TurnInc;
        Counter = 0;
        if abs(Turn) > 90
            TurnInc = -TurnInc;
        end
    end
end

== matlab function RoboBoat_SLAM_6_29/Main FSM/Start Speed/Gate Find and Through1/Find/MATLAB Function1 ==
  data: Dist input; Angles input; X input; Y input; Heading input; found output; Goal output; DesiredHeading output
function [found, Goal, DesiredHeading] = SpeedGate(Dist,Angles,X,Y,Heading)
%Written by Anderson Lebbad on May 29, 2015
%Last Edited by:

%This function sends theboat forward until a landmark is found, then it
%navigates towards the right of it.

persistent goalX goalY Found initialHeading change
if isempty(goalX)
    goalX = X;
    goalY = Y;
    Found = 0;
    initialHeading = Heading;
    change = 10;
end

DesiredHeading = Heading;
DistM = Dist./100;
dodgeWidth = 3;

if Found == 0
    if DistM(2) ~= 0
        %If two objects are found, set goal between the two
        w = (DistM(1)*sin(Angles(1)) + DistM(2)*sin(Angles(2)*pi/180)) / 2;
        h = (DistM(1)*cos(Angles(1)) + DistM(2)*sin(Angles(2)*pi/180)) / 2;
        goalX = X + h*cos(Heading) - w*sin(Heading);
        goalY = Y + h*sin(Heading) + w*cos(Heading);
        Found = 1;
    elseif DistM(1) ~= 0
        %If one object is found, set goal dodgewidth to the right of it
        w = DistM(1)*sin(Angles(1)) + dodgeWidth;
        h = DistM(1)*cos(Angles(1));
        goalX = X + h*cos(Heading) - w*sin(Heading);
        goalY = Y + h*sin(Heading) + w*cos(Heading);
        Found = 1;
    else
        %If no objects are found, search. Scan 30 degrees to left and right
        %of initial heading.
        DesiredHeading = Heading + change;
        if abs(DesiredHeading - initialHeading) > 30
            change = -change;
            DesiredHeading = Heading + change;
        end
    end
end

Goal = [goalX, goalY];
found = Found;

end

== matlab function RoboBoat_SLAM_6_29/Main FSM/Obstacle Navigation1/Enter Gate/Gate 2 (White & White)/MATLAB Function ==
  data: Prob input; RPM output; ColorID input; Dist input; Ang input; CurrentHeading input; GPSLat input; GPSLong input; Timer input; DesiredHeading output; gateGPS output
function [RPM,DesiredHeading,gateGPS] = navigation(Prob,ColorID,Dist,Ang,CurrentHeading,GPSLat,GPSLong,Timer)

% Function performs one buoy navigation through the start speed gates. If
% no buoys are found by the LIDAR/Vision assembly then an incremented
% turning algorithm is executed to turn by 10 degrees per increment up to 
% 90 degrees either way of the inital heading

% Written by Edward Zhu


persistent LockHeading TimeLastFound Counter Turn TurnInc gateLat gateLong

if isempty(LockHeading) && isempty(TimeLastFound) && isempty(Counter) && isempty(Turn) && isempty(TurnInc)
    LockHeading = CurrentHeading;
    TimeLastFound = 0;
    Counter = 0;
    TurnInc = 30;
    Turn = TurnInc;
    gateLat = 0;
    gateLong = 0;
end
Distance = Dist/100;
BoatWidth = 0.75;
Buffer = atan(2*BoatWidth/Distance);

RedOffset = Ang + Buffer;
WhiteOffset = Ang - Buffer;

R = 6378137;

CurLat = (floor(GPSLat/100)+mod(GPSLat,100)/60)*pi/180;
CurLong = (ceil(GPSLong/100)-mod(-GPSLong,100)/60)*pi/180;

gateHeading = (mod(CurrentHeading - Ang, 360))*pi/180;

if ColorID == 1 && Prob > 0.9
    DesiredHeading = mod(CurrentHeading - RedOffset, 360);
    RPM = 2000;
    GateFound = 1;
    TimeLastFound = Timer;
    gateLat =  asin(sin(CurLat)*cos(Distance/R) + cos(CurLat)*sin(Distance/R)*cos(gateHeading))*180/pi;
    gateLong = (CurLong + atan2(sin(gateHeading)*sin(Distance/R)*cos(CurLat),cos(Distance/R)-sin(CurLat)*sin(gateLat)))*180/pi;
elseif ColorID == 2 && Prob > 0.9
    DesiredHeading = mod(CurrentHeading - WhiteOffset, 360);
    RPM = 2000;
    GateFound = 1;
    TimeLastFound = Timer;
    gateLat =  asin(sin(CurLat)*cos(Distance/R) + cos(CurLat)*sin(Distance/R)*cos(gateHeading))*180/pi;
    gateLong = (CurLong + atan2(sin(gateHeading)*sin(Distance/R)*cos(CurLat),cos(Distance/R)-sin(CurLat)*sin(gateLat)))*180/pi;
else
    DesiredHeading = CurrentHeading;
    RPM = 0;
    GateFound = 0;
end

gateGPS = [gateLat gateLong];
TimeNoBuoys = Timer - TimeLastFound;

if GateFound == 0 && TimeNoBuoys > 15
    RPM = 0;
    DesiredHeading = mod(LockHeading - Turn, 360);
    HeadingDiff = DesiredHeading - CurrentHeading;
    gateGPS = [gateLat gateLong];
    
    if HeadingDiff > 180
        HeadingDiff = HeadingDiff - 360;
    elseif HeadingDiff < -180
        HeadingDiff = HeadingDiff + 360;
    end
    
    if HeadingDiff < 3
        Counter = Counter + 1;
    else
        Counter = 0;
    end
    
    if Counter >= 15
        Turn = Turn + TurnInc;
        Counter = 0;
        if abs(Turn) > 90
            TurnInc = -TurnInc;
        end
    end
end
